simulink model "PI_Controller"  (R2020b)
settings: Solver=VariableStepAuto  StartTime=0.0  StopTime=10.0  RelTol=1e-3
values from neighbouring files (symbols this model uses):
  Ki = 0.185    [variables.m]
  Kp = 2.28    [variables.m]
  Ts = 0.01    [variables.m]
settings Model: DataDictionary=Cruise_Control.sldd  Creator=Akshata Ashok  LastModifiedBy=Akshata Ashok

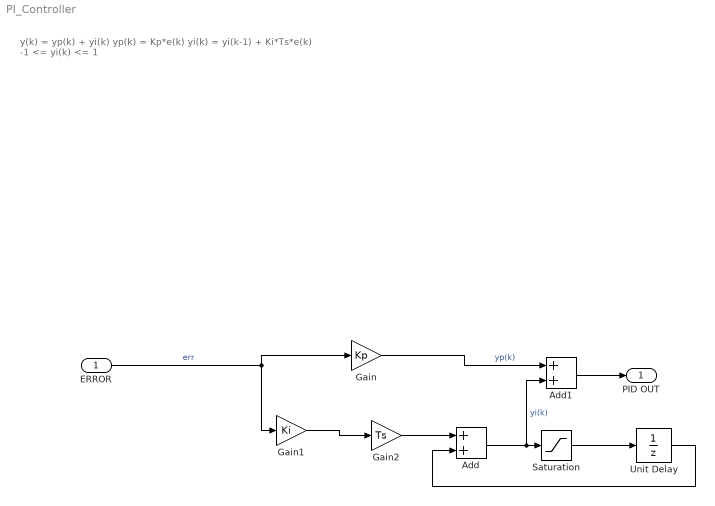
== system PI_Controller ==
  note: y(k) = yp(k) + yi(k)
      |
      | yp(k) = Kp*e(k)
      |
      | yi(k) = yi(k-1) + Ki*Ts*e(k)
      |
      | -1 <= yi(k) <= 1
  ERROR : Inport  OutDataTypeStr=double  PortDimensions=1  SampleTime=0
  Add : Sum
  Add1 : Sum
  Gain : Gain  Gain=Kp
  Gain1 : Gain  Gain=Ki
  Gain2 : Gain  Gain=Ts
  Saturation : Saturate  UpperLimit=1  LowerLimit=-1
  Unit Delay : UnitDelay  SampleTime=-1  HasFrameUpgradeWarning=on
  PID OUT : Outport  OutDataTypeStr=double  PortDimensions=1  SampleTime=0
  wires:
  ERROR/1 -> Gain/1, Gain1/1  "err"
  Unit Delay/1 -> Add/2
  Saturation/1 -> Unit Delay/1
  Gain/1 -> Add1/1  "yp(k)"
  Gain1/1 -> Gain2/1
  Add1/1 -> PID OUT/1
  Gain2/1 -> Add/1
  Add/1 -> Saturation/1, Add1/2  "yi(k)"
